simulink model "SMC"  (Simulink 10.0)
settings: Solver=VariableStepAuto  StartTime=0.0  StopTime=60  FixedStep=0.02  RelTol=1e-3
model workspace (MAT data in the model file):
  table = [0.138956796593 0.189366832537 0.239777858744 0.290189875214 0.340602881948 0.391016878945 0.441431866206 0.491829747338 0.544679911093 0.601596169389 0.662578522228 0.727626969608 ... (2244 elements, 33x68)]
  table_2 = [0.48 0.587855357616 0.711975093401 0.852359207353 1 1 1 1 1 1 1 1 ... (442 elements, 13x34)]
libraries: simulink x2, Solver_SF x1
settings Model: Creator=JHD  LastModifiedBy=JHD  SimulationMode=accelerator
settings SolverCC: ZeroCrossAlgorithm=Adaptive  AlgebraicLoopSolver=LineSearch
settings DataIOCC: SaveFormat=Dataset  ReturnWorkspaceOutputs=on
settings OptimizationCC: LifeSpan=auto
settings DebuggingCC: UnderspecifiedInitializationDetection=Simplified  MergeDetectMultiDrivingBlocksExec=error  SFUnexpectedBacktrackingDiag=error  SFNoUnconditionalDefaultTransitionDiag=error  SFExecutionAtInitializationDiag=warning  ArithmeticOperatorsInVariantConditions=error
settings HardwareCC: ProdBitPerPointer=64  ProdBitPerSizeT=64  ProdBitPerPtrDiffT=64  ProdLargestAtomicFloat=Float  ProdIntDivRoundTo=Zero  ProdEndianess=LittleEndian  ProdWordSize=64  ProdHWDeviceType=Intel->x86-64 (Windows64)
settings ModelReferenceCC: PropagateSignalLabelsOutOfModel=on
settings SFSimCC: SimUseLocalCustomCode=on  CustomCodeUndefinedFunction=FilterOut
settings RTWCC: RTWUseLocalCustomCode=on
settings CodeAppCC: StateflowObjectComments=off
settings GRTTargetCC: TargetLangStandard=C99 (ISO)  CombineOutputUpdateFcns=on  GRTInterface=off
settings ConfigComp: CovMetricSettings=dwe  CovHtmlReporting=off  CovSaveCumulativeToWorkspaceVar=off  CovSaveSingleToWorkspaceVar=off

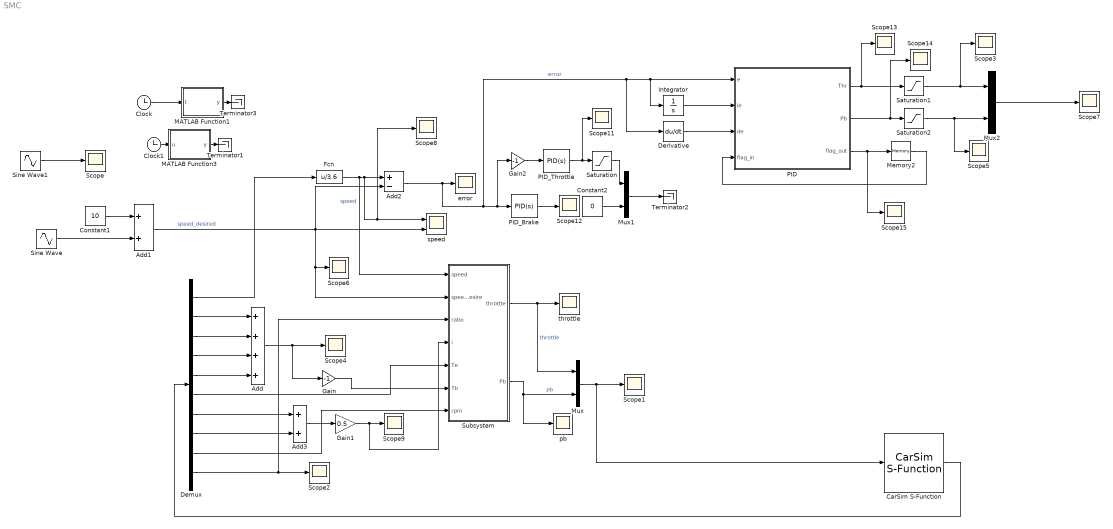
== system SMC ==
  Add : Sum  Inputs=++++
  Add1 : Sum
  Add2 : Sum  Inputs=+-
  Add3 : Sum
  CarSim S-Function : Solver_SF/CarSim S-Function  Priority=1  SIMFILE=simfile.sim
  Clock : Clock
  Clock1 : Clock
  Constant1 : Constant  Value=10
  Constant2 : Constant  Value=0
  Demux : Demux  Outputs=10
  Derivative : Derivative
  Fcn : Fcn  Expr=u/3.6
  Gain : Gain  Gain=-1
  Gain1 : Gain  Gain=0.5
  Gain2 : Gain  Gain=-1
  Integrator : Integrator
  MATLAB Function1 : MATLAB Function  TreatAsAtomicUnit=on
  MATLAB Function3 : MATLAB Function  TreatAsAtomicUnit=on
  Memory2 : Memory
  Mux : Mux  Inputs=2
  Mux1 : Mux  Inputs=2
  Mux2 : Mux  Inputs=2
  PID : MATLAB Function  TreatAsAtomicUnit=on
  PID_Brake : simulink/Continuous/PID Controller  Controller=PID  Form=Parallel  TimeDomain=Continuous-time  SampleTime=-1  IntegratorMethod=Forward Euler  FilterMethod=Forward Euler  ControllerParametersSource=internal  P=1  I=0  D=0  UseFilter=on  N=100  TunerSelectOption=Transfer Function Based (PID Tuner App)  InitialConditionSource=internal  InitialConditionForIntegrator=0  InitialConditionForFilter=0  DifferentiatorICPrevScaledInput=0  ExternalReset=none  TrackingMode=off  Kt=1  LimitOutput=off  UpperSaturationLimit=inf  LowerSaturationLimit=-inf  LinearizeAsGain=on  AntiWindupMode=none  Kb=1  POutMin=[]  POutMax=[]  IOutMin=[]  IOutMax=[]  DOutMin=[]  DOutMax=[]  NOutMin=[]  NOutMax=[]  SumOutMin=[]  SumOutMax=[]  SaturationOutMin=[]  SaturationOutMax=[]  PParamMin=[]  PParamMax=[]  IParamMin=[]  IParamMax=[]  DParamMin=[]  DParamMax=[]  NParamMin=[]  NParamMax=[]  KbParamMin=[]  KbParamMax=[]  KtParamMin=[]  KtParamMax=[]  KbOutMin=[]  KbOutMax=[]  KtOutMin=[]  KtOutMax=[]  IntegratorOutMin=[]  IntegratorOutMax=[]  FilterOutMin=[]  FilterOutMax=[]  SumI1OutMin=[]  SumI1OutMax=[]  SumI2OutMin=[]  SumI2OutMax=[]  SumI3OutMin=[]  SumI3OutMax=[]  SumI4OutMin=[]  SumI4OutMax=[]  SumDOutMin=[]  SumDOutMax=[]  DifferentiatorOutMin=[]  DifferentiatorOutMax=[]  FilterDiffOutCoefMin=[]  FilterDiffOutCoefMax=[]  ReciprocalOutMin=[]  ReciprocalOutMax=[]  SumDenOutMin=[]  SumDenOutMax=[]  SumNumOutMin=[]  SumNumOutMax=[]  DivideOutMin=[]  DivideOutMax=[]  IntegratorContinuousStateAttributes=''  IntegratorStateMustResolveToSignalObject=off  IntegratorRTWStateStorageClass=Auto  FilterContinuousStateAttributes=''  FilterStateMustResolveToSignalObject=off  FilterRTWStateStorageClass=Auto  ParallelPVariant=InternalParameters  IdealPVariant=Disabled  IVariant=InternalParameters  DVariant=InternalParameters  IntegratorVariant=Continuous  SatVariant=Disabled  AWVariant=Passthrough  PCopyVariant=Disabled  TRVariant=Disabled  FdbkBlocksVariant=Forward  IdealPFdbkVariant=Disabled  SatFdbkVariant=Disabled  DerivativeFilterVariant=ContFilter  NVariant=InternalParameters  NCopyVariant=Disabled  FilterICVariant=InternalICsFilter  IntegratorICVariant=InternalICs  ExternalResetVariant=Disabled  TRSumVariant=Passthrough  SumFdbkVariant=Disabled  SumVariant=Sum_PID
  PID_Throttle : simulink/Continuous/PID Controller  Controller=PID  Form=Parallel  TimeDomain=Continuous-time  SampleTime=-1  IntegratorMethod=Forward Euler  FilterMethod=Forward Euler  ControllerParametersSource=internal  P=400  I=0  D=0  UseFilter=on  N=100  TunerSelectOption=Transfer Function Based (PID Tuner App)  InitialConditionSource=internal  InitialConditionForIntegrator=0  InitialConditionForFilter=0  DifferentiatorICPrevScaledInput=0  ExternalReset=none  TrackingMode=off  Kt=1  LimitOutput=off  UpperSaturationLimit=inf  LowerSaturationLimit=-inf  LinearizeAsGain=on  AntiWindupMode=none  Kb=1  POutMin=[]  POutMax=[]  IOutMin=[]  IOutMax=[]  DOutMin=[]  DOutMax=[]  NOutMin=[]  NOutMax=[]  SumOutMin=[]  SumOutMax=[]  SaturationOutMin=[]  SaturationOutMax=[]  PParamMin=[]  PParamMax=[]  IParamMin=[]  IParamMax=[]  DParamMin=[]  DParamMax=[]  NParamMin=[]  NParamMax=[]  KbParamMin=[]  KbParamMax=[]  KtParamMin=[]  KtParamMax=[]  KbOutMin=[]  KbOutMax=[]  KtOutMin=[]  KtOutMax=[]  IntegratorOutMin=[]  IntegratorOutMax=[]  FilterOutMin=[]  FilterOutMax=[]  SumI1OutMin=[]  SumI1OutMax=[]  SumI2OutMin=[]  SumI2OutMax=[]  SumI3OutMin=[]  SumI3OutMax=[]  SumI4OutMin=[]  SumI4OutMax=[]  SumDOutMin=[]  SumDOutMax=[]  DifferentiatorOutMin=[]  DifferentiatorOutMax=[]  FilterDiffOutCoefMin=[]  FilterDiffOutCoefMax=[]  ReciprocalOutMin=[]  ReciprocalOutMax=[]  SumDenOutMin=[]  SumDenOutMax=[]  SumNumOutMin=[]  SumNumOutMax=[]  DivideOutMin=[]  DivideOutMax=[]  IntegratorContinuousStateAttributes=''  IntegratorStateMustResolveToSignalObject=off  IntegratorRTWStateStorageClass=Auto  FilterContinuousStateAttributes=''  FilterStateMustResolveToSignalObject=off  FilterRTWStateStorageClass=Auto  ParallelPVariant=InternalParameters  IdealPVariant=Disabled  IVariant=InternalParameters  DVariant=InternalParameters  IntegratorVariant=Continuous  SatVariant=Disabled  AWVariant=Passthrough  PCopyVariant=Disabled  TRVariant=Disabled  FdbkBlocksVariant=Forward  IdealPFdbkVariant=Disabled  SatFdbkVariant=Disabled  DerivativeFilterVariant=ContFilter  NVariant=InternalParameters  NCopyVariant=Disabled  FilterICVariant=InternalICsFilter  IntegratorICVariant=InternalICs  ExternalResetVariant=Disabled  TRSumVariant=Passthrough  SumFdbkVariant=Disabled  SumVariant=Sum_PID
  Saturation : Saturate  UpperLimit=300  LowerLimit=-50
  Saturation1 : Saturate  UpperLimit=1  LowerLimit=0
  Saturation2 : Saturate  UpperLimit=2  LowerLimit=0
  Scope{,1..9,11..15} (15 alike) : Scope
  Sine Wave : Sin  Amplitude=6  Frequency=0.3  Phase=7.5*pi  SampleTime=0
  Sine Wave1 : Sin  Amplitude=6  Frequency=0.3  SampleTime=0
  Subsystem : Subsystem
  Terminator1 : Terminator
  Terminator2 : Terminator
  Terminator3 : Terminator
  error : Scope
  pb : Scope
  speed : Scope  NumInputPorts=2
  throttle : Scope
  wires:
  Constant1/1 -> Add1/1
  Demux/8 -> Add3/2
  Fcn/1 -> Subsystem/1(speed), Add2/1, Scope8/1, speed/1  "speed"
  Demux/7 -> Add3/1
  Sine Wave/1 -> Add1/2
  Add2/1 -> Derivative/1, Integrator/1, PID/1(e), Gain2/1, PID_Brake/1, error/1  "error"
  Demux/6 -> Subsystem/5(Te)
  Demux/5 -> Add/4
  Demux/4 -> Add/3
  Demux/3 -> Add/2
  Demux/1 -> Fcn/1
  CarSim S-Function/1 -> Demux/1
  Add/1 -> Gain/1, Scope4/1
  Clock/1 -> MATLAB Function1/1(t)
  Add1/1 -> Add2/2, speed/2, Subsystem/2(speed_desire), Scope6/1  "speed_desired"
  Demux/9 -> Subsystem/7(rpm)
  Add3/1 -> Gain1/1
  Gain2/1 -> PID_Throttle/1
  PID_Throttle/1 -> Scope11/1, Saturation/1
  PID_Brake/1 -> Scope12/1
  Mux1/1 -> Terminator2/1
  Saturation/1 -> Mux1/1
  Constant2/1 -> Mux1/2
  Derivative/1 -> PID/3(de)
  Integrator/1 -> PID/2(ie)
  PID/1(Thr) -> Saturation1/1, Scope13/1
  PID/2(Pb) -> Saturation2/1, Scope14/1
  PID/3(flag_out) -> Scope15/1, Memory2/1
  Memory2/1 -> PID/4(flag_in)
  Mux2/1 -> Scope7/1
  Saturation1/1 -> Scope3/1, Mux2/1
  Mux/1 -> CarSim S-Function/1, Scope1/1
  Saturation2/1 -> Scope5/1, Mux2/2
  Subsystem/1(throttle) -> Mux/1, throttle/1  "throttle"
  Subsystem/2(Pb) -> pb/1, Mux/2  "pb"
  Gain/1 -> Subsystem/6(Tb)
  Clock1/1 -> MATLAB Function3/1(u)
  MATLAB Function3/1(y) -> Terminator1/1
  Demux/2 -> Add/1
  Demux/10 -> Scope2/1, Subsystem/3(ratio)
  Gain1/1 -> Subsystem/4(i), Scope9/1
  MATLAB Function1/1(y) -> Terminator3/1
  Sine Wave1/1 -> Scope/1

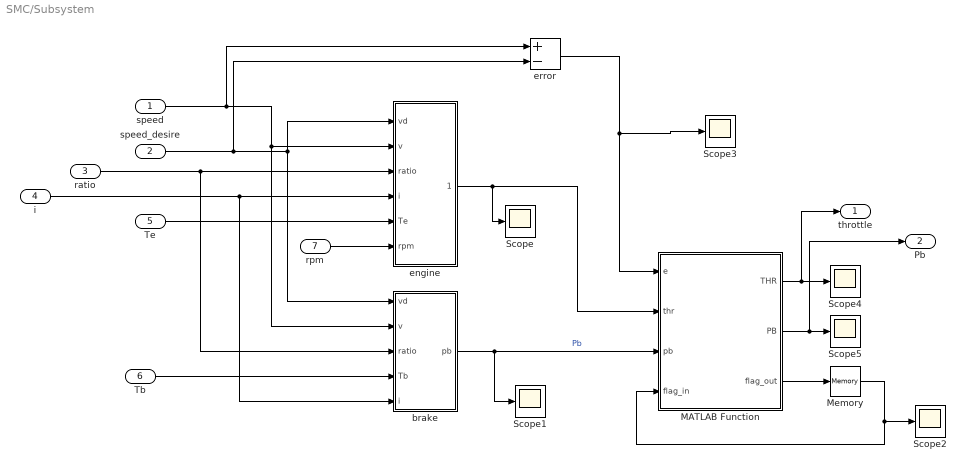
== system SMC/Subsystem ==
  speed : Inport
  speed_desire : Inport  Port=2
  ratio : Inport  Port=3
  i : Inport  Port=4
  Te : Inport  Port=5
  Tb : Inport  Port=6
  rpm : Inport  Port=7
  MATLAB Function : MATLAB Function  TreatAsAtomicUnit=on
  Memory : Memory
  Scope{,1..5} (6 alike) : Scope
  brake : Subsystem
  engine : Subsystem
  error : Sum  Inputs=+-
  throttle : Outport
  Pb : Outport  Port=2
  wires:
  speed/1 -> error/1, brake/2(v), engine/2(v)
  brake/1(pb) -> Scope1/1, MATLAB Function/3(pb)  "Pb"
  speed_desire/1 -> error/2, brake/1(vd), engine/1(vd)
  engine/1(throttle) -> Scope/1, MATLAB Function/2(thr)
  ratio/1 -> brake/3(ratio), engine/3(ratio)
  i/1 -> brake/5(i), engine/4(i)
  Te/1 -> engine/5(Te)
  Tb/1 -> brake/4(Tb)
  rpm/1 -> engine/6(rpm)
  MATLAB Function/3(flag_out) -> Memory/1
  Memory/1 -> MATLAB Function/4(flag_in), Scope2/1
  error/1 -> Scope3/1, MATLAB Function/1(e)
  MATLAB Function/1(THR) -> throttle/1, Scope4/1
  MATLAB Function/2(PB) -> Pb/1, Scope5/1

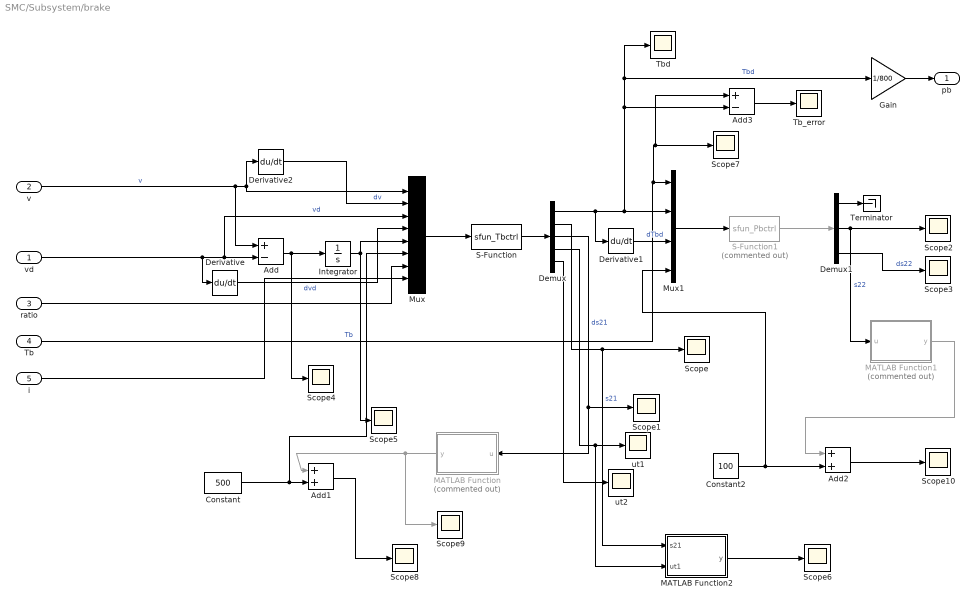
== system SMC/Subsystem/brake ==
  vd : Inport
  v : Inport  Port=2
  ratio : Inport  Port=3
  Tb : Inport  Port=4
  i : Inport  Port=5
  Add : Sum  Inputs=+-
  Add1 : Sum
  Add2 : Sum
  Add3 : Sum  Inputs=+-
  Constant : Constant  Value=500
  Constant2 : Constant  Value=100
  Demux : Demux  Outputs=5
  Demux1 : Demux  Outputs=3
  Derivative : Derivative
  Derivative1 : Derivative
  Derivative2 : Derivative
  Gain : Gain  Gain=1/800
  Integrator : Integrator
  MATLAB Function : MATLAB Function  Commented=on  TreatAsAtomicUnit=on
  MATLAB Function1 : MATLAB Function  Commented=on  TreatAsAtomicUnit=on
  MATLAB Function2 : MATLAB Function  TreatAsAtomicUnit=on
  Mux : Mux  Inputs=8
  Mux1 : Mux
  S-Function : S-Function  FunctionName=sfun_Tbctrl  SFunctionDeploymentMode=off  EnableBusSupport=off
  S-Function1 : S-Function  Commented=on  FunctionName=sfun_Pbctrl  SFunctionDeploymentMode=off  EnableBusSupport=off
  Scope{,1..10} (11 alike) : Scope
  Tb_error : Scope
  Tbd : Scope
  Terminator : Terminator
  ut1 : Scope
  ut2 : Scope
  pb : Outport
  wires:
  S-Function1/1 -> Demux1/1
  Add/1 -> Scope4/1, Integrator/1
  Derivative/1 -> Mux/4  "dvd"
  Demux/1 -> Derivative1/1, Add3/2, Tbd/1, Gain/1, Mux1/2  "Tbd"
  vd/1 -> Mux/3, Add/2, Derivative/1  "vd"
  Mux/1 -> S-Function/1
  Derivative1/1 -> Mux1/3  "dTbd"
  Derivative2/1 -> Mux/2  "dv"
  Integrator/1 -> Mux/5, Scope5/1
  S-Function/1 -> Demux/1
  Mux1/1 -> S-Function1/1
  v/1 -> Add/1, Derivative2/1, Mux/1  "v"
  ratio/1 -> Mux/7
  Tb/1 -> Add3/1, Scope7/1, Mux1/1  "Tb"
  Demux/2 -> Scope/1, MATLAB Function2/1(s21)  "s21"
  Demux/3 -> Scope1/1, MATLAB Function/1(u)  "ds21"
  Demux1/3 -> Scope3/1  "ds22"
  Demux1/2 -> MATLAB Function1/1(u), Scope2/1  "s22"
  Constant/1 -> Mux/6, Add1/2
  Add1/1 -> Scope8/1
  MATLAB Function/1(y) -> Scope9/1, Add1/1
  MATLAB Function1/1(y) -> Add2/1
  Constant2/1 -> Mux1/4, Add2/2
  Add2/1 -> Scope10/1
  i/1 -> Mux/8
  Demux/4 -> MATLAB Function2/2(ut1), ut1/1
  Demux/5 -> ut2/1
  Add3/1 -> Tb_error/1
  Demux1/1 -> Terminator/1
  Gain/1 -> pb/1
  MATLAB Function2/1(y) -> Scope6/1

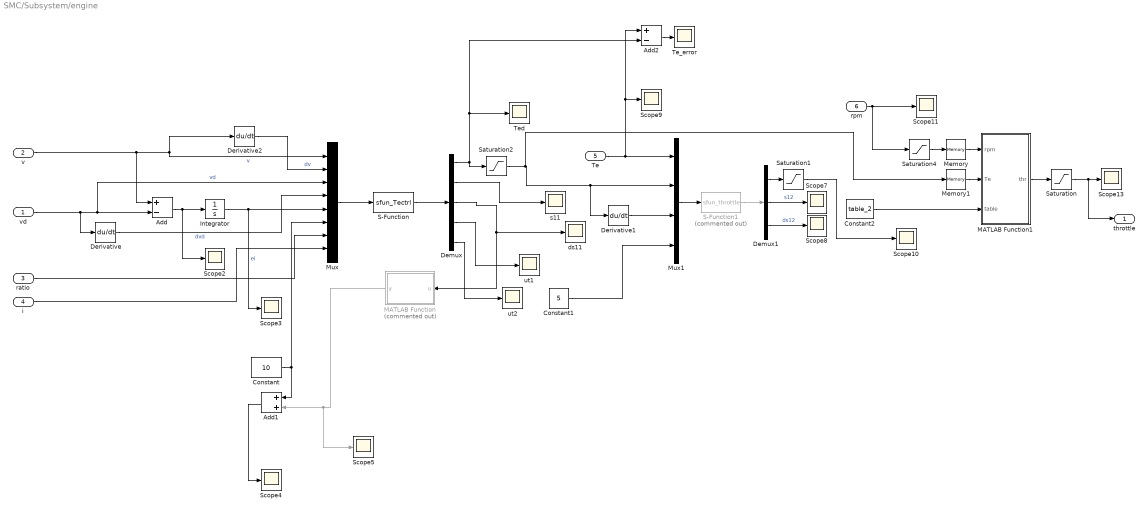
== system SMC/Subsystem/engine ==
  vd : Inport
  v : Inport  Port=2
  ratio : Inport  Port=3
  i : Inport  Port=4
  Te : Inport  Port=5
  rpm : Inport  Port=6
  Add : Sum  Inputs=+-
  Add1 : Sum
  Add2 : Sum  Inputs=+-
  Constant : Constant  Value=10
  Constant1 : Constant  Value=5
  Constant2 : Constant  Value=table_2
  Demux : Demux  Outputs=5
  Demux1 : Demux  Outputs=3
  Derivative : Derivative
  Derivative1 : Derivative
  Derivative2 : Derivative
  Integrator : Integrator
  MATLAB Function : MATLAB Function  Commented=on  TreatAsAtomicUnit=on
  MATLAB Function1 : MATLAB Function  TreatAsAtomicUnit=on
  Memory : Memory
  Memory1 : Memory
  Mux : Mux  Inputs=8
  Mux1 : Mux
  S-Function : S-Function  FunctionName=sfun_Tectrl  SFunctionDeploymentMode=off  EnableBusSupport=off
  S-Function1 : S-Function  Commented=on  FunctionName=sfun_throttle  SFunctionDeploymentMode=off  EnableBusSupport=off
  Saturation : Saturate  UpperLimit=1  LowerLimit=0
  Saturation1 : Saturate  UpperLimit=250  LowerLimit=0
  Saturation2 : Saturate  UpperLimit=250  LowerLimit=0
  Saturation4 : Saturate  UpperLimit=6700  LowerLimit=0
  Scope{2..5,7..11,13} (10 alike) : Scope
  Te_error : Scope
  Ted : Scope
  ds11 : Scope
  s11 : Scope
  ut1 : Scope
  ut2 : Scope
  throttle : Outport
  wires:
  S-Function/1 -> Demux/1
  Integrator/1 -> Scope3/1, Mux/5  "ei"
  Derivative2/1 -> Mux/2  "dv"
  Mux/1 -> S-Function/1
  vd/1 -> Add/2, Mux/3, Derivative/1  "vd"
  Derivative/1 -> Mux/4  "dvd"
  Add/1 -> Scope2/1, Integrator/1
  v/1 -> Mux/1, Derivative2/1, Add/1  "v"
  ratio/1 -> Mux/7
  Demux/2 -> s11/1
  Demux/3 -> ds11/1, MATLAB Function/1(u)
  Constant/1 -> Mux/6, Add1/1
  Add1/1 -> Scope4/1
  MATLAB Function/1(y) -> Add1/2, Scope5/1
  i/1 -> Mux/8
  Mux1/1 -> S-Function1/1
  Te/1 -> Scope9/1, Add2/1, Mux1/1
  Constant1/1 -> Mux1/4
  Derivative1/1 -> Mux1/3
  S-Function1/1 -> Demux1/1
  Demux1/2 -> Scope7/1  "s12"
  Demux1/3 -> Scope8/1  "ds12"
  MATLAB Function1/1(thr) -> Saturation/1
  Demux1/1 -> Saturation1/1
  Constant2/1 -> MATLAB Function1/3(table)
  Saturation/1 -> throttle/1, Scope13/1
  Saturation1/1 -> Scope10/1
  Saturation4/1 -> Memory/1
  rpm/1 -> Saturation4/1, Scope11/1
  Saturation2/1 -> Memory1/1, Mux1/2, Derivative1/1
  Memory/1 -> MATLAB Function1/1(rpm)
  Memory1/1 -> MATLAB Function1/2(Te)
  Add2/1 -> Te_error/1
  Demux/1 -> Saturation2/1, Add2/2, Ted/1
  Demux/4 -> ut1/1
  Demux/5 -> ut2/1

== matlab function Subsystem/brake/MATLAB Function ==
  data: u input double; y output double
function y = fcn(u)

k_u=10;
k_y=5;
u=u/k_u;
mf=[-4/3 -1 -2/3 -1/3 0 1/3 2/3 1 4/3];
N=7;
y1=zeros(N,1);
y2=zeros(N,1);
s1=zeros(N,1);
for i=1:N
    y1(i)=trimf_smc(u,mf(i),mf(1+i),mf(2+i));
    s1(i)=(2/3-3*y1(i))*y1(i);
    y2(i)=s1(i)*mf(N+2-i);
end
s1_sum=0;
y2_sum=0;
for i=1:N
    s1_sum=s1_sum+s1(i);
    y2_sum=y2_sum+y2(i);
end
y=y2_sum/s1_sum*k_y;

if u>1||u<-1
    y=0;
end
end

== matlab function Subsystem/engine/MATLAB Function ==
  data: u input double; y output double
function y = fcn(u)

k_u=10;
k_y=5;
u=u/k_u;
mf=[-4/3 -1 -2/3 -1/3 0 1/3 2/3 1 4/3];
N=7;
y1=zeros(N,1);
y2=zeros(N,1);
s1=zeros(N,1);
for i=1:N
    y1(i)=trimf_smc(u,mf(i),mf(1+i),mf(2+i));
    s1(i)=(2/3-3*y1(i))*y1(i);
    y2(i)=s1(i)*mf(N+2-i);
end
s1_sum=0;
y2_sum=0;
for i=1:N
    s1_sum=s1_sum+s1(i);
    y2_sum=y2_sum+y2(i);
end
y=y2_sum/s1_sum*k_y;

if u>1||u<-1
    y=0;
end
end

== matlab function Subsystem/brake/MATLAB Function1 ==
  data: u input double; y output double
function y = fcn(u)

k_u=150;
k_y=5;
u=u/k_u;
mf=[-4/3 -1 -2/3 -1/3 0 1/3 2/3 1 4/3];
N=7;
y1=zeros(N,1);
y2=zeros(N,1);

for i=1:N
    y1(i)=trimf_smc(u,mf(i),mf(1+i),mf(2+i));
    y2(i)=mf(N+2-i);
end

[~,index]=max(y1);
y=y2(index)*k_y;

if u>1||u<-1
    y=0;
end

end

== matlab function Subsystem/brake/MATLAB Function2 ==
  data: s21 input double; y output double; ut1 input double
function y = fcn(s21, ut1)

ut2=20*sign(s21);
%ut2=k21*sat(s21);
ut = (ut1+ut2)/800;
if ut<0
    ut=0;
end
if ut>2
    ut=2;
end
y = ut;


function m=sat(s)
k=0.05;
d=abs(s/k);
if d<=1
    m=s/k;
else
    m=sign(s/k);
end

== matlab function MATLAB Function1 ==
  data: t input double; y output double
function y = fcn(t)

t1 = 8;
t2 = 6;
k1 = 6;
k2 = 4;
T = 60;
k3 = 7.5;
k4 = 5;

if t<t1
    y = 5;
elseif t<pi * k1 + t1
    y = sin((t-pi/2*k1-t1) * 1/k1) * k3 + 5+k3;
elseif t<T-pi*k2-t2
    y= 5 + 2*k3;
elseif t<T-t2
    y = cos(1/k2*(t + pi*k2 -T +t2)) * k4 + 5+2*k3-k4;
else
    y = 5+2*k3-2*k4;
end

== matlab function PID ==
  data: e input double; Thr output double; Pb output double; ie input double; de input double; flag_in input double; flag_out output double
function [Thr, Pb, flag_out]= fcn(e, ie, de, flag_in)
kp_thr = -0.3;
ki_thr = -0.05;  % -1
kd_thr = 0;

kp_brk = 4;
ki_brk = 0.1;
kd_brk = 0;

thr = kp_thr * e + ki_thr * ie + kd_thr * de;
pb = kp_brk * e + ki_brk * ie + kd_brk * de;

switch flag_in
    case 0
        if e < -0.2
            Thr = thr;
            Pb = 0;
            flag_out = 1;
        else
            Pb = pb;
            Thr = 0;
            flag_out = 0;
        end
    otherwise
         if e > 0.2
             Pb = pb;
             Thr = 0;
             flag_out = 0;
         else
             Thr = thr;
             Pb = 0;
             flag_out = 1;
         end
end

== matlab function Subsystem/engine/MATLAB Function1 ==
  data: rpm input double; thr output double; Te input double; table input double
function thr = fcn(rpm, Te, table)

% x=0:100:6700;
% y=-67.65:10:252.35;

x=0:200:6700;
y=0:20:250;

z=table;
thr=interp2(x,y,z,rpm,Te);

== matlab function Subsystem/MATLAB Function ==
  data: e input double; THR output double; thr input double; pb input double; flag_in input double; PB output double; flag_out output double
function [THR, PB, flag_out]= fcn(e, thr, pb, flag_in)

switch flag_in
    case 0
        if thr>0.067 && e < -0.03
            THR = thr;
            PB = 0;
            flag_out = 1;
        else
            PB = pb;
            THR = 0;
            flag_out = 0;
        end
    otherwise
         if pb>0.02 && e > 0.03
             PB = pb;
             THR = 0;
             flag_out = 0;
         else
             THR = thr;
             PB = 0;
             flag_out = 1;
         end
end

== matlab function MATLAB Function3 ==
  data: u input double; y output double
function y = fcn(u)

k1 = 10;
T = 60;
k2 = 15;

if u<pi/2 * k1
    y = sin(u * 1/k1) * k2;
else
    if u<T-pi/2*k1
        y=1 * k2;
    else
        y = sin(1/k1*(u - T + pi*k1)) * k2;
    end
end
